simulink model "gm_lorenz_model_interface"  (R2018a)
settings: Solver=FixedStepAuto  StartTime=0.0  StopTime=inf  RelTol=1e-3  EnableMultiTasking=on
libraries: alterasoclib x5, simulink_extras x1
settings Model: SimulationMode=external  Creator=labuser  LastModifiedBy=labuser
settings SolverCC: ConcurrentTasks=on  PositivePriorityOrder=on
settings OptimizationCC: BlockReduction=off  ConditionallyExecuteInputs=off  EnhancedBackFolding=on  PassReuseOutputArgsAs=Individual arguments  MaxStackSize=64  OptimizeBlockOrder=speed  DifferentSizesBufferReuse=on  OptimizationCustomize=off
settings DebuggingCC: AlgebraicLoopMsg=error  ParameterTunabilityLossMsg=error
settings HardwareCC: ProdBitPerPointer=32  ProdBitPerSizeT=32  ProdBitPerPtrDiffT=32  ProdLargestAtomicInteger=Long  ProdLargestAtomicFloat=Double  ProdWordSize=32  ProdHWDeviceType=ARM Compatible->ARM Cortex  TargetBitPerPointer=64  TargetBitPerSizeT=64  TargetBitPerPtrDiffT=64  TargetLongLongMode=on  TargetIntDivRoundTo=Zero  TargetEndianess=LittleEndian  TargetWordSize=64  TargetHWDeviceType=Custom Processor->MATLAB Host Computer
settings SFSimCC: MATLABDynamicMemAlloc=off
settings RTWCC: SystemTargetFile=ert.tlc  HardwareBoard=Altera Cyclone V SoC development kit  TLCOptions="-aInlineSetEventsForThisBaseRateFcn=TLC_FALSE -aSuppressMultiTaskScheduler=TLC_FALSE  -aRateBasedStepFcn=0"  TemplateMakefile=ert_default_tmf  GenerateReport=on  Toolchain=ARM Development Studio Altera Edition (DS-5 AE)  IncludeHyperlinkInReport=on  LaunchReport=on  GenerateTraceInfo=on  GenerateTraceReport=on  GenerateTraceReportSl=on  GenerateTraceReportSf=on  GenerateTraceReportEml=on
settings CodeAppCC: ForceParamTrailComments=on  IgnoreCustomStorageClasses=off  OperatorAnnotations=on  SimulinkDataObjDesc=on  SFDataObjDesc=on  InsertBlockDesc=on

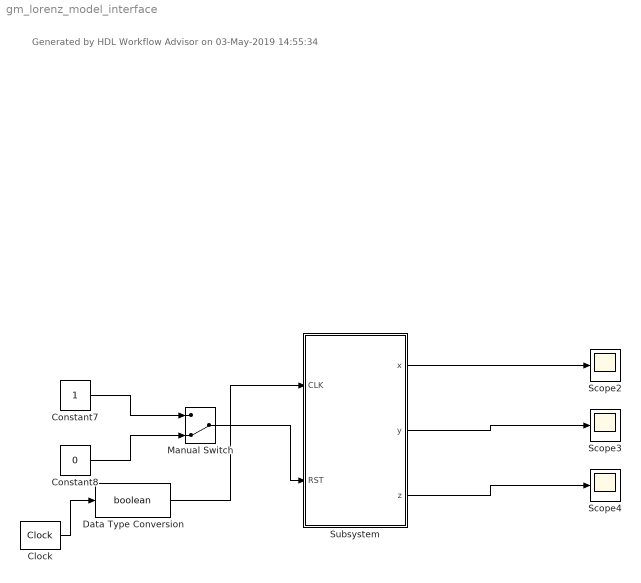
== system gm_lorenz_model_interface ==
  note: Generated by HDL Workflow Advisor on 03-May-2019 14:55:34
  Clock : simulink_extras/Flip Flops/Clock  period=0.0001
  Constant7 : Constant  OutDataTypeStr=boolean  SampleTime=-1
  Constant8 : Constant  Value=0  OutDataTypeStr=boolean  SampleTime=-1
  Data Type Conversion : DataTypeConversion  OutDataTypeStr=boolean
  Manual Switch : ManualSwitch  CurrentSetting=0
  Scope2 : Scope
  Scope3 : Scope
  Scope4 : Scope
  Subsystem : Subsystem  TreatAsAtomicUnit=on  mask(AXI4-Lite/AXI4 Interface){}
      mask help:
      | This is an automatically generated subsystem block.
      | This contains the AXI interface blocks that communicate with the Subsystem_ip IPCore generated from lorenz_model/Subsystem subsystem.
      mask Display: disp(sprintf('Altera SoC \nAXI Interface'));
  wires:
  Data Type Conversion/1 -> Subsystem/1(CLK)
  Clock/1 -> Data Type Conversion/1
  Manual Switch/1 -> Subsystem/2(RST)
  Constant8/1 -> Manual Switch/2
  Constant7/1 -> Manual Switch/1
  Subsystem/2(y) -> Scope3/1
  Subsystem/3(z) -> Scope4/1
  Subsystem/1(x) -> Scope2/1

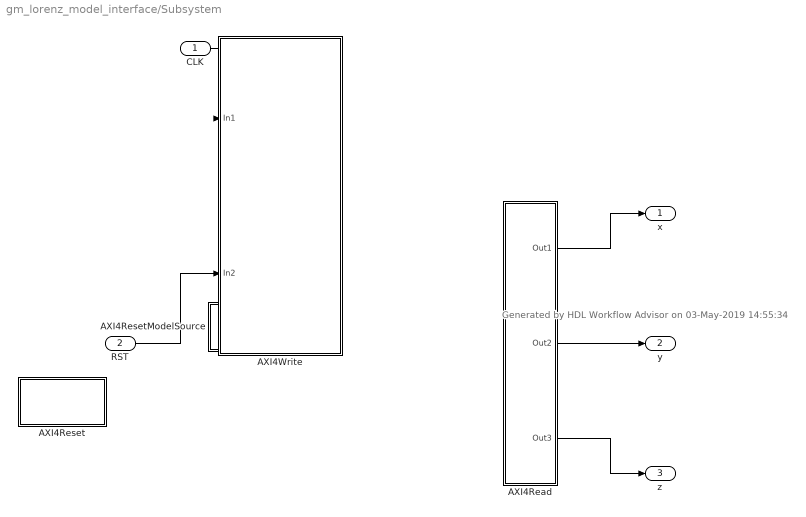
== system gm_lorenz_model_interface/Subsystem ==
  note: Generated by HDL Workflow Advisor on 03-May-2019 14:55:34
  CLK : Inport  OutDataTypeStr=boolean
  RST : Inport  Port=2  OutDataTypeStr=boolean
  AXI4Read : Subsystem  Priority=10
  AXI4Reset : Subsystem  mask(System Start){ShowInLibBrowser=0}
      mask prompts: ShowInLibBrowser "Simulink:masks:CustCodeMaskParam1_MP"
      settings: CopyFcn=cccopyfcn(gcb)  OpenFcn=ccopenfcn('System Start Function')
      mask Help: eval('feval(''rtwprivate'',''rtwhelpview'',''rtw_sys_start_block'')');
      mask Display: disp('System\nStart');
  AXI4ResetModelSource : Subsystem  mask(Model Source){ShowInLibBrowser=0}
      mask prompts: ShowInLibBrowser "Simulink:masks:CustCodeMaskParam1_MP"
      settings: CopyFcn=cccopyfcn(gcb)  OpenFcn=ccopenfcn('Model Source')
      mask Help: eval('feval(''rtwprivate'',''rtwhelpview'',''rtw_model_source_block'')');
      mask Display: disp('Model\nSource');
  AXI4Write : Subsystem  Priority=1
  x : Outport  OutDataTypeStr=fixdt(1,27,20)
  y : Outport  Port=2  OutDataTypeStr=fixdt(1,27,20)
  z : Outport  Port=3  OutDataTypeStr=fixdt(1,27,20)
  wires:
  CLK/1 -> AXI4Write/1(In1)
  RST/1 -> AXI4Write/2(In2)
  AXI4Read/1(Out1) -> x/1
  AXI4Read/2(Out2) -> y/1
  AXI4Read/3(Out3) -> z/1

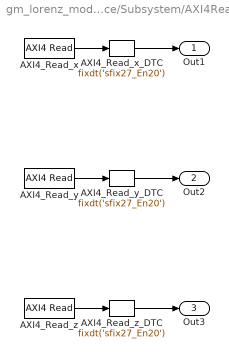
== system gm_lorenz_model_interface/Subsystem/AXI4Read ==
  AXI4_Read_x : alterasoclib/AXI4 Read  Priority=2  DeviceName=/dev/mwipcore  RegisterOffset=hex2dec('108')  DataType=uint32  DataLength=1  SampleTime=-1  BlockPlatform=ALTERASOC
      settings: SourceProductName=Embedded Coder Support Package for Intel SoC Devices  SourceProductBaseCode=EC_ALTERA_SOC
  AXI4_Read_x_DTC : DataTypeConversion  OutDataTypeStr=fixdt('sfix27_En20')  ConvertRealWorld=Stored Integer (SI)
  AXI4_Read_y : alterasoclib/AXI4 Read  Priority=3  DeviceName=/dev/mwipcore  RegisterOffset=hex2dec('104')  DataType=uint32  DataLength=1  SampleTime=-1  BlockPlatform=ALTERASOC
      settings: SourceProductName=Embedded Coder Support Package for Intel SoC Devices  SourceProductBaseCode=EC_ALTERA_SOC
  AXI4_Read_y_DTC : DataTypeConversion  OutDataTypeStr=fixdt('sfix27_En20')  ConvertRealWorld=Stored Integer (SI)
  AXI4_Read_z : alterasoclib/AXI4 Read  Priority=4  DeviceName=/dev/mwipcore  RegisterOffset=hex2dec('100')  DataType=uint32  DataLength=1  SampleTime=-1  BlockPlatform=ALTERASOC
      settings: SourceProductName=Embedded Coder Support Package for Intel SoC Devices  SourceProductBaseCode=EC_ALTERA_SOC
  AXI4_Read_z_DTC : DataTypeConversion  OutDataTypeStr=fixdt('sfix27_En20')  ConvertRealWorld=Stored Integer (SI)
  Out1 : Outport
  Out2 : Outport  Port=2
  Out3 : Outport  Port=3
  wires:
  AXI4_Read_x/1 -> AXI4_Read_x_DTC/1
  AXI4_Read_z/1 -> AXI4_Read_z_DTC/1
  AXI4_Read_y/1 -> AXI4_Read_y_DTC/1
  AXI4_Read_z_DTC/1 -> Out3/1
  AXI4_Read_y_DTC/1 -> Out2/1
  AXI4_Read_x_DTC/1 -> Out1/1

== system gm_lorenz_model_interface/Subsystem/AXI4Reset ==

== system gm_lorenz_model_interface/Subsystem/AXI4ResetModelSource ==

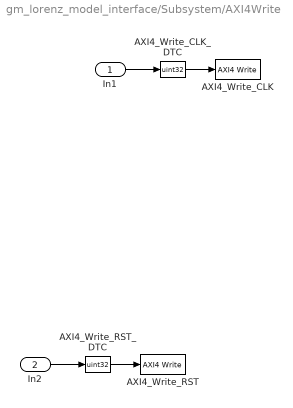
== system gm_lorenz_model_interface/Subsystem/AXI4Write ==
  In1 : Inport
  In2 : Inport  Port=2
  AXI4_Write_CLK : alterasoclib/AXI4 Write  Priority=1  DeviceName=/dev/mwipcore  RegisterOffset=hex2dec('10C')  BlockPlatform=ALTERASOC
      settings: SourceProductName=Embedded Coder Support Package for Intel SoC Devices  SourceProductBaseCode=EC_ALTERA_SOC
  AXI4_Write_CLK_DTC : DataTypeConversion  OutDataTypeStr=uint32  ConvertRealWorld=Stored Integer (SI)
  AXI4_Write_RST : alterasoclib/AXI4 Write  Priority=2  DeviceName=/dev/mwipcore  RegisterOffset=hex2dec('110')  BlockPlatform=ALTERASOC
      settings: SourceProductName=Embedded Coder Support Package for Intel SoC Devices  SourceProductBaseCode=EC_ALTERA_SOC
  AXI4_Write_RST_DTC : DataTypeConversion  OutDataTypeStr=uint32  ConvertRealWorld=Stored Integer (SI)
  wires:
  AXI4_Write_CLK_DTC/1 -> AXI4_Write_CLK/1
  In1/1 -> AXI4_Write_CLK_DTC/1
  In2/1 -> AXI4_Write_RST_DTC/1
  AXI4_Write_RST_DTC/1 -> AXI4_Write_RST/1
